simulink model "ModelAgriAuto"  (R2022a)
settings: Solver=FixedStepAuto  StartTime=0.0  StopTime=6240  FixedStep=0.05  MaxStep=0.1  RelTol=1e-3
model workspace (MAT data in the model file):
  PlowHectare = 1.925
values from neighbouring files (symbols this model uses):
  C_rate = 3    [start_function.m]
  Compaction = 0    [start_function.m]
  CyclesIn = CyclesIn+CyclesOut(end)    [start_function.m]
  Degradation = 2    [start_function.m]
  FailRate = 29700000    [start_function.m]
  FieldEff = 0.8    [start_function.m]
  ForceCorrVar = 0.85    [start_function.m]
  Fuel = 3    [start_function.m]
  Mass = 10550    [start_function.m]
  n = n+1    (= 2)    [start_function.m]
  v_field = 5    [start_function.m]
  Weather_crit = 3    [start_function.m]
  WorkingHours = 10    [start_function.m]
undefined symbols (not defined in the file or in its folder): Battery, BatteryNo, Charger, ChargerNo, DField, m, Power, Soil, TractorNo, Year
libraries: simulink x2
(part 1 of 3)
settings Model: Creator=osov0001  LastModifiedBy=osov0001
settings SolverCC: AlgebraicLoopSolver=LineSearch
settings DataIOCC: ExternalInput=[Power, Battery, Charger]  SaveFormat=Array  SaveOutput=off  DSMLogging=off  ReturnWorkspaceOutputs=off
settings DebuggingCC: UnconnectedInputMsg=warning  UnconnectedOutputMsg=warning  UnconnectedLineMsg=warning  SFMachineParentedDataDiag=warning  ArithmeticOperatorsInVariantConditions=warning
settings SFSimCC: SimUseLocalCustomCode=off  CustomCodeUndefinedFunction=UseInterfaceOnly
settings RTWCC: RTWUseLocalCustomCode=off

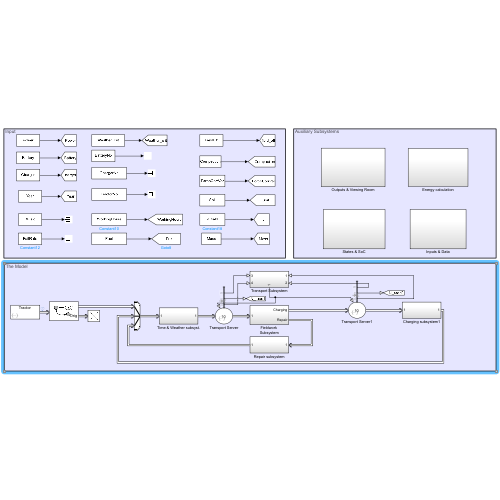
[thumbnail: Simulink's stored preview of the top-level diagram]
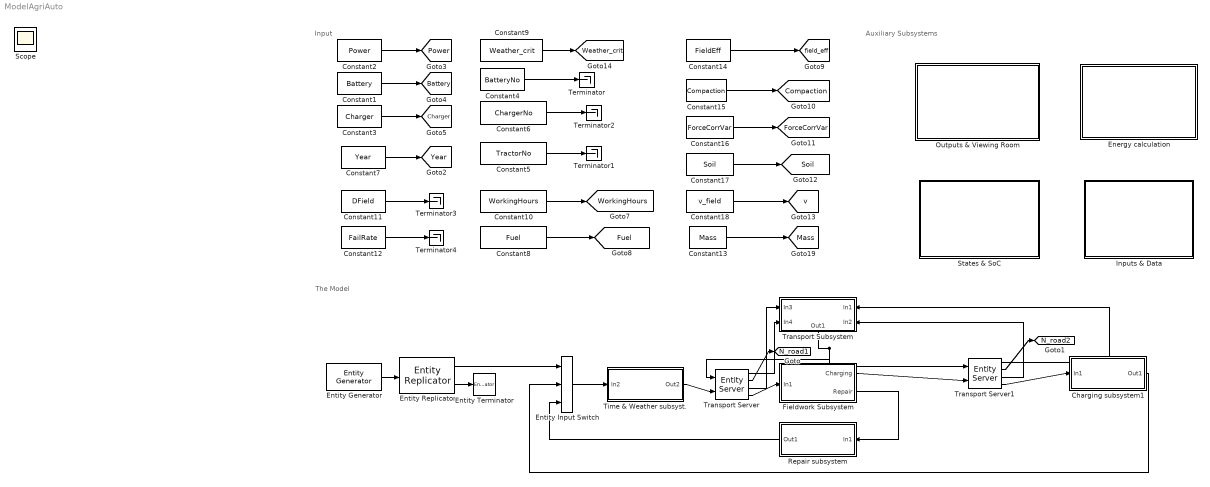
== system ModelAgriAuto ==
  note: The Model
  note: Input
  note: Auxiliary Subsystems
  Charging subsystem1 : Subsystem
  Constant1 : Constant  Value=Battery
  Constant10 : Constant  Value=WorkingHours
  Constant11 : Constant  Value=DField
  Constant12 : Constant  Value=FailRate
  Constant13 : Constant  Value=Mass
  Constant14 : Constant  Value=FieldEff
  Constant15 : Constant  Value=Compaction
  Constant16 : Constant  Value=ForceCorrVar
  Constant17 : Constant  Value=Soil
  Constant18 : Constant  Value=v_field
  Constant2 : Constant  Value=Power
  Constant3 : Constant  Value=Charger
  Constant4 : Constant  Value=BatteryNo
  Constant5 : Constant  Value=TractorNo
  Constant6 : Constant  Value=ChargerNo
  Constant7 : Constant  Value=Year
  Constant8 : Constant  Value=Fuel
  Constant9 : Constant  Value=Weather_crit
  Energy calculation : Subsystem
  Entity Input Switch : EntityInputSwitch  InputPortMessageModes=m,m,m  OutputPortMessageModes=m  NumberInputPorts=3
      settings: InputPortMap=u1,u2,u3
  Entity Generator : EntityGenerator  OutputPortMessageModes=m  Period=inf  GenerateAction=|  AttributeName=SoC|RoadTime|RoF  AttributeInitialValue=1|1|1  EntityType=Structured  EntityTypeName=Tractor
      | entity.SoC=1;
      | entity.RoF=1;
  Entity Replicator : EntityReplicator  InputPortMessageModes=m  OutputPortMessageModes=m,m  ReplicasDepartFrom=Single output port  NumberReplicas=TractorNo  HoldOriginalEntityUntilAllReplicasDepart=on
  Entity Terminator : EntityTerminator  InputPortMessageModes=m
  Fieldwork Subsystem : Subsystem
  Inputs & Data : Subsystem  Tag=INPUTS
  Outputs & Viewing Room : Subsystem
  Repair subsystem : Subsystem
  States & SoC : Subsystem
  Terminator{,1..4} (5 alike) : Terminator
  Time & Weather subsyst. : Subsystem
  Transport Server : EntityServer  InputPortMessageModes=n,m  OutputPortMessageModes=n,n,n,m  Capacity=10  ServiceTimeSource=Signal port  ServiceTimeAttributeName=RoadTime  ServiceCompleteAction=entity.SoC=entity.SoC-0.025;  NumberEntitiesDeparted=on  NumberEntitiesInBlock=on  AverageWait=on
      settings: InputPortMap=u0,u2  OutputPortMap=o0,o1,o4,o9
  Transport Server1 : EntityServer  InputPortMessageModes=n,m  OutputPortMessageModes=n,n,n,m  Capacity=10  ServiceTimeSource=Signal port  ServiceTimeAttributeName=RoadTime  ServiceCompleteAction=entity.SoC=entity.SoC-0.025;  NumberEntitiesDeparted=on  NumberEntitiesInBlock=on  AverageWait=on
      settings: InputPortMap=u0,u2  OutputPortMap=o0,o1,o4,o9
  Transport Subsystem : Subsystem
      settings: PortSchema="{\"entries\":[{\"content\":{\"sides\":[{\"content\":{\"connectorIds\":[\"In1\",\"In2\"]},\"type\":\"ConnectorPlacement.EquallySpacedRectSide\",\"uuid\":\"550b19fe-7368-4b75-be55-a28990181de4\"},{\"content\":{\"connectorIds\":[\"In3\",\"In4\"],\"side\":\"RIGHT\"},\"type\":\"ConnectorPlacement.EquallySpacedRectSide\",\"uuid\":\"f910dc23-d412-48e8-995a-8c291cfed89a\"},{\"content\":{\"connectorIds\":[],\"side\":\"TOP\"},\"type\":\"ConnectorPlacement.EquallySpacedRectSide\",\"uuid\":\"9035d057-4d0f-475c-8836-3d54a9fb5317\"},{\"content\":{\"connectorIds\":[\"Out1\"],\"side\":\"BOTTOM\"},\"type\":\"ConnectorPlacement.EquallySpacedRectSide\",\"uuid\":\"2f36d4ef-6e1b-49a3-b865-e90f10116552\"}]},\"type\":\"ConnectorPlacement.EquallySpacedConnector\",\"uuid\":\"6736081e-50e9-4bc7-8291-962b989661d1\"}],\"packageUris\":[\"http://schema.mathworks.com/mf0/Connector/R2020b\"],\"version\":\"1.0\"}"
  Scope : Scope
  tag scope: Battery=global, Charger=global, Compaction=global, ForceCorrVar=global, Fuel=global, Mass=global, N_road1=global, N_road2=global, Power=global, Soil=global, Weather_crit=global, WorkingHours=global, Year=global, field_eff=global, v=global
  wires:
  Entity Replicator/2 -> Entity Terminator/1
  Entity Generator/1 -> Entity Replicator/1
  Fieldwork Subsystem/1(Charging) -> Transport Server1/2
  Transport Server1/4 -> Charging subsystem1/1(In1)
  Charging subsystem1/1(Out1) -> Entity Input Switch/2
  Repair subsystem/1(Out1) -> Entity Input Switch/3
  Entity Input Switch/1 -> Time & Weather subsyst./1(In2)
  Fieldwork Subsystem/2(Repair) -> Repair subsystem/1(In1)
  Constant1/1 -> [Battery]
  Constant3/1 -> [Charger]
  Constant6/1 -> Terminator2/1
  Constant5/1 -> Terminator1/1
  Constant4/1 -> Terminator/1
  Constant7/1 -> [Year]
  Constant9/1 -> [Weather_crit]
  Transport Server1/3 -> Transport Subsystem/2(In2)
  Transport Server1/1 -> Transport Subsystem/1(In1)
  Entity Replicator/1 -> Entity Input Switch/1
  Transport Server/2 -> [N_road1]
  Transport Server1/2 -> [N_road2]
  Constant10/1 -> [WorkingHours]
  Constant8/1 -> [Fuel]
  Transport Server/4 -> Fieldwork Subsystem/1(In1)
  Constant11/1 -> Terminator3/1
  Time & Weather subsyst./1(Out2) -> Transport Server/2
  Constant2/1 -> [Power]
  Constant12/1 -> Terminator4/1
  Constant13/1 -> [Mass]
  Constant14/1 -> [field_eff]
  Constant15/1 -> [Compaction]
  Constant16/1 -> [ForceCorrVar]
  Constant17/1 -> [Soil]
  Constant18/1 -> [v]
  Transport Subsystem/1(Out1) -> Transport Server/1, Transport Server1/1
  Transport Server/3 -> Transport Subsystem/3(In3)
  Transport Server/1 -> Transport Subsystem/4(In4)

== system ModelAgriAuto/Charging subsystem1 ==
  note: Tid att ladda [h]
  In1 : Inport
  Add3 : Sum  Inputs=+++
  Add4 : Sum
  Add5 : Sum
  Avg queue length : Display
  Avg wait time [h] : Display
  Battery exchange system : Subsystem
  "Charger type and power calculation subsystem " : Subsystem
  Display : DisplayBlock  LabelPosition=Hide  Format=long
  Display2 : Display
  Energy Calculation : Subsystem
  Entity Input Switch1 : EntityInputSwitch  InputPortMessageModes=m,m  OutputPortMessageModes=m
  Entity Output Switch1 : EntityOutputSwitch  InputPortMessageModes=m,m  OutputPortMessageModes=m,m  SwitchingCriterion=From control port  SwitchAttributeName=Attribute1
      settings: InputPortMap=u0,u1
  Entity Queue1 : Queue  InputPortMessageModes=m  OutputPortMessageModes=n,n,m  AverageWait=on  AverageQueueLength=on
      settings: OutputPortMap=o2,o3,o5
  Product1 : Product  Inputs=3
  Product2 : Product
  To Workspace : ToWorkspace  VariableName=TC  SampleTime=1
      settings: Save2DSignal=2-D array (concatenate along first dimension)
  To Workspace1 : ToWorkspace  VariableName=Q_wait_avg  SampleTime=1
  To Workspace3 : ToWorkspace  VariableName=TQ  SampleTime=1
      settings: Save2DSignal=2-D array (concatenate along first dimension)
  Traditional charging/refueling : Subsystem
  Out1 : Outport  VectorParamsAs1DForOutWhenUnconnected=off
  tag scope: Charger_time=global, T_Charge=global
  wires:
  Entity Queue1/3 -> Entity Output Switch1/2
  In1/1 -> Entity Queue1/1
  "Charger type and power calculation subsystem "/1(Charger time) -> [Charger_time]
  Entity Output Switch1/1 -> Traditional charging/refueling/1(In1)
  "Charger type and power calculation subsystem "/2(Charger type) -> Entity Output Switch1/1
  Product1/1 -> Add3/2
  Entity Queue1/1 -> To Workspace1/1, Product1/1, Avg wait time [h]/1  "Avg waiting time [h]"
  Add4/1 -> Display2/1, [T_Charge]
  Entity Queue1/2 -> Avg queue length/1, Product1/2  "Avg queue length [no.]"
  Entity Input Switch1/1 -> Out1/1
  Product2/1 -> Add5/1
  [Charge_no] -> Product1/3
  [Change_no] -> Product2/1
  Traditional charging/refueling/4(Charge time) -> Add5/2
  Add5/1 -> Add4/2, To Workspace/1
  Add3/1 -> To Workspace3/1, Add4/1
  Traditional charging/refueling/2(Queue time) -> Add3/3
  Traditional charging/refueling/1(Out1) -> Entity Input Switch1/1
  Traditional charging/refueling/3(Entities departed) -> Energy Calculation/1(In1)
  Entity Output Switch1/2 -> Battery exchange system/1(In2)
  Battery exchange system/1(Out2) -> Entity Input Switch1/2
  Battery exchange system/2(Out1) -> Product2/2
  Battery exchange system/3(Out3) -> Add3/1

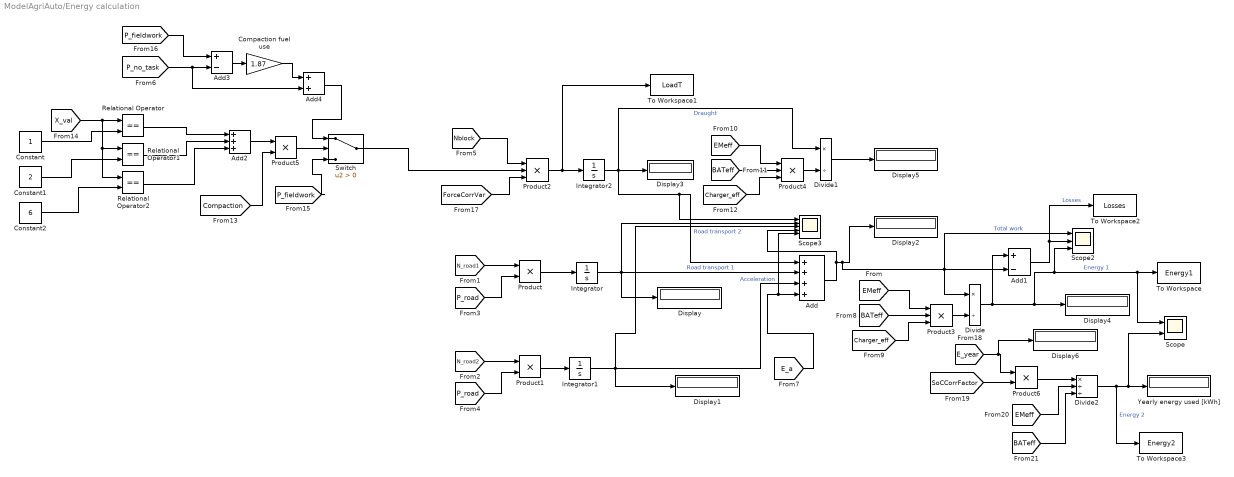
== system ModelAgriAuto/Energy calculation ==
  Add : Sum  Inputs=++++
  Add1 : Sum  Inputs=+-
  Add2 : Sum  Inputs=+++
  Add3 : Sum  Inputs=+-
  Add4 : Sum
  Compaction fuel use : Gain  Gain=1.87
  Constant : Constant
  Constant1 : Constant  Value=2
  Constant2 : Constant  Value=6
  Display{,1..6} (7 alike) : Display
  Divide : Product  Inputs=*/
  Divide1 : Product  Inputs=*/
  Divide2 : Product  Inputs=*//
  Integrator : Integrator
  Integrator1 : Integrator
  Integrator2 : Integrator
  Product{,1,5..6} (4 alike) : Product
  Product2 : Product  Inputs=3
  Product3 : Product  Inputs=3
  Product4 : Product  Inputs=3
  Relational Operator : RelationalOperator  Operator===  OutDataTypeStr=boolean  RndMeth=Simplest  InputSameDT=off
  Relational Operator1 : RelationalOperator  Operator===  OutDataTypeStr=boolean  RndMeth=Simplest  InputSameDT=off
  Relational Operator2 : RelationalOperator  Operator===  OutDataTypeStr=boolean  RndMeth=Simplest  InputSameDT=off
  Scope : Scope  NumInputPorts=2
  Scope2 : Scope  NumInputPorts=3
  Scope3 : Scope  NumInputPorts=5
  Switch : Switch  Criteria=u2 > Threshold  SaturateOnIntegerOverflow=off  InputSameDT=off
  To Workspace : ToWorkspace  VariableName=Energy1  SampleTime=1
  To Workspace1 : ToWorkspace  VariableName=LoadT  SampleTime=0.5
      settings: Save2DSignal=2-D array (concatenate along first dimension)
  To Workspace2 : ToWorkspace  VariableName=Losses  SampleTime=1
  To Workspace3 : ToWorkspace  VariableName=Energy2  SampleTime=1
  Yearly energy used [kWh] : Display
  wires:
  [N_road1] -> Product/1
  [P_road] -> Product/2
  [P_road] -> Product1/2
  [N_road2] -> Product1/1
  Product/1 -> Integrator/1
  Product1/1 -> Integrator1/1
  Integrator/1 -> Add/2, Scope3/2, Display/1  "Road transport 1"
  Integrator1/1 -> Add/3, Display1/1, Scope3/3  "Road transport 2"
  Add/1 -> Display2/1, Add1/2, Divide/1, Scope2/1, Scope3/4  "Total work"
  [Nblock] -> Product2/1
  [E_a] -> Scope3/5, Add/4  "Acceleration"
  Divide/1 -> Add1/1, Scope2/3, Scope/1, To Workspace/1, Display4/1  "Energy 1"
  [Charger_eff] -> Product3/3
  [BATeff] -> Product3/2
  [EMeff] -> Product3/1
  Product3/1 -> Divide/2
  [Charger_eff] -> Product4/3
  [EMeff] -> Product4/1
  Product4/1 -> Divide1/2
  [BATeff] -> Product4/2
  Integrator2/1 -> Display3/1, Scope3/1, Add/1, Divide1/1  "Draught"
  Divide1/1 -> Display5/1
  Product2/1 -> Integrator2/1, To Workspace1/1
  Add1/1 -> Scope2/2, To Workspace2/1  "Losses"
  Relational Operator/1 -> Add2/1
  Relational Operator1/1 -> Add2/2
  Relational Operator2/1 -> Add2/3
  [X_val] -> Relational Operator2/1, Relational Operator1/1, Relational Operator/1
  Constant/1 -> Relational Operator/2
  Constant1/1 -> Relational Operator1/2
  Constant2/1 -> Relational Operator2/2
  Add2/1 -> Product5/1
  [Compaction] -> Product5/2
  Product5/1 -> Switch/2
  [P_fieldwork] -> Switch/3
  Switch/1 -> Product2/2
  [P_fieldwork] -> Add3/1
  [P_no_task] -> Add4/2, Add3/2
  Add3/1 -> Compaction fuel use/1
  Compaction fuel use/1 -> Add4/1
  Add4/1 -> Switch/1
  [ForceCorrVar] -> Product2/3
  Divide2/1 -> To Workspace3/1, Scope/2, Yearly energy used [kWh]/1  "Energy 2"
  Product6/1 -> Divide2/1
  [BATeff] -> Divide2/3
  [E_year] -> Display6/1, Product6/1
  [EMeff] -> Divide2/2
  [SoCCorrFactor] -> Product6/2

== system ModelAgriAuto/Fieldwork Subsystem ==
  In1 : Inport
  Active working time [days] : Display
  Entity Output Switch : EntityOutputSwitch  InputPortMessageModes=m  OutputPortMessageModes=m,m  SwitchingCriterion=From attribute  SwitchAttributeName=entity.RoF
  Entity Gate : EntityGate  InputPortMessageModes=m,m  OutputPortMessageModes=m  OpenGateAtSimulationStart=on
  Entity Queue : Queue  InputPortMessageModes=m  OutputPortMessageModes=n,n,m  Capacity=10  NumberEntitiesDeparted=on  AverageWait=on
      settings: OutputPortMap=o0,o2,o5
  Failure check : EntityServer  InputPortMessageModes=m  OutputPortMessageModes=m  Capacity=1  ServiceTimeValue=0.01  ServiceCompleteAction=|
      | M=(FailRate);
      | x=randi (M);
      | 
      | % if-loop determined by Rate- of-failure
      | if x>=M;
      |     entity.RoF=2;
      | else
      |     entity.RoF=1;
      | end
  Field Subsystem : Subsystem
  "Fieldwork time subsystem " : Subsystem
  FieldworkServer : EntityServer  InputPortMessageModes=n,m  OutputPortMessageModes=n,n,n,m  Capacity=10  ServiceTimeSource=Signal port  ServiceTimeValue=3.843  NumberEntitiesDeparted=on  NumberEntitiesInBlock=on  AverageWait=on
      settings: InputPortMap=u0,u2  OutputPortMap=o0,o1,o4,o9
  Message Send : Send  OutputPortMessageModes=m
  No. of tractor-trips : Display
  Null Server : EntityServer  InputPortMessageModes=m  OutputPortMessageModes=n,m  Capacity=1  ServiceTimeValue=0.0001  NumberEntitiesDeparted=on
      settings: OutputPortMap=o0,o9
  Product : Product
  Product1 : Product
  Saturation : Saturate  UpperLimit=WorkingHours  LowerLimit=0
  Scope : Scope
  To Workspace : ToWorkspace  VariableName=Hectares  SampleTime=1
  To Workspace1 : ToWorkspace  VariableName=Field  SampleTime=1
  To Workspace2 : ToWorkspace  VariableName=Task  SampleTime=1
  To Workspace3 : ToWorkspace  VariableName=WorkTime  SampleTime=1
  h to days : Gain  Gain=1/24
  Charging : Outport  VectorParamsAs1DForOutWhenUnconnected=off
  Repair : Outport  Port=2  VectorParamsAs1DForOutWhenUnconnected=off
  tag scope: Field=global, Nblock=global, T_Wait=global, T_Work=global, Trips=global
  wires:
  In1/1 -> Null Server/1
  FieldworkServer/3 -> Product/1
  Null Server/2 -> Entity Queue/1
  Field Subsystem/4(Out5) -> To Workspace/1  "H out total"
  Field Subsystem/1(Out2) -> Message Send/1
  Field Subsystem/3(Out4) -> To Workspace2/1  "Task number"
  Message Send/1 -> Entity Gate/1
  Field Subsystem/2(Out3) -> [Field], To Workspace1/1  "Field number"
  FieldworkServer/1 -> Product/2
  Null Server/1 -> [Trips], No. of tractor-trips/1
  Product1/1 -> [T_Wait]
  Entity Queue/1 -> Product1/2
  Entity Queue/2 -> Product1/1
  Entity Queue/3 -> Entity Gate/2
  FieldworkServer/2 -> [Nblock], Field Subsystem/1(N_block)
  Entity Output Switch/1 -> FieldworkServer/2
  Entity Output Switch/2 -> Repair/1
  Failure check/1 -> Entity Output Switch/1
  Entity Gate/1 -> Failure check/1
  Product/1 -> h to days/1, [T_Work], To Workspace3/1
  h to days/1 -> Active working time [days]/1
  "Fieldwork time subsystem "/1(Out1) -> Saturation/1
  Saturation/1 -> Scope/1, FieldworkServer/1
  FieldworkServer/4 -> Charging/1

== system ModelAgriAuto/Inputs & Data ==
  note: Fuel & Driveline inputs
  note: Weather inputs
  note: Charger inputs
  note: Field, soil and crop rotation inputs
  Battery and driveline inputs : Subsystem
  Charging inputs : Subsystem
  Field inputs : Subsystem
  "Fuel/mode selection " : Subsystem
  Weather Inputs : Subsystem

== system ModelAgriAuto/Outputs & Viewing Room ==
  note: Time distribution
  note: Periods:
      |
      | Spring period: 0 - 1512 h
      |
      | Growing period: 1513 - 2208 h
      |
      | Summer period: 2209 - 2976 h
      |
      | Growing and harvest period: 2978 - 4104 h
      |
      | Fall period: 4105-5600 h
  note: Operation order:
      |
      | 1: -
      | 2: Harrow / Harvning
      | 3: Fert. Spreading / Gödsling
      | 4: Harrow / Harvning
      | 5: Sowing / Sådd
      | 6: Roller packing / Vältning
      | ------
      | 7: Fert. Spreading / Gödsling
      | 8: Fert. Spreading / Gödsling
      | 9: Pesticide Spreading / Växtskydd
      | ------
      | (Harvest / Skörd)
      | 10: Cultivation / Stubbning
      | 11: Cultivation / Sladdning
      | 12: Roller packing / Vältning
      | 13: Fert. Spreading / Gödsling
      | 14: Harrow / Harvning
      | 15: Harrow / Harvning
      | 16: Sowing / Sådd
      | 17: Plowing / Plöjning
  Active time in field [days] : DisplayBlock  LabelPosition=Hide  Format=long
  Dashboard Scope : DashboardScope  Ymin=0  Ymax=100
  Favourable weather [%] : DisplayBlock  LabelPosition=Hide  Format=long
  No. of charges : DisplayBlock  LabelPosition=Hide  Format=long
  No. of repairs : DisplayBlock  LabelPosition=Hide  Format=long
  No. of trips : DisplayBlock  LabelPosition=Hide  Format=long
  Rate of failure [%] : DisplayBlock  LabelPosition=Hide  Format=long
  Time Management Subsystem : Subsystem
  Time required (alt) [days/yr] : DisplayBlock  LabelPosition=Hide  Format=long
  Yearly energy consumption [kWh] : DisplayBlock  LabelPosition=Hide  Format=shortE

== system ModelAgriAuto/Repair subsystem ==
  In1 : Inport
  Display1 : Display
  Gain : Gain  Gain=100
  No. of repairs : Display
  Product1 : Product  Inputs=**
  Product2 : Product  Inputs=*/
  Repair : EntityServer  InputPortMessageModes=n,m  OutputPortMessageModes=n,m  Capacity=1  ServiceTimeSource=Signal port  ServiceTimeValue=24  NumberEntitiesDeparted=on
      settings: InputPortMap=u0,u2  OutputPortMap=o0,o9
  Repair time : Constant  Value=24
  Out1 : Outport  VectorParamsAs1DForOutWhenUnconnected=off
  tag scope: RoF=global, T_Repair=global
  wires:
  Repair/1 -> Product2/1, Product1/2, No. of repairs/1
  In1/1 -> Repair/2
  Repair/2 -> Out1/1
  Product2/1 -> [RoF]
  [Trips] -> Product2/2
  Repair time/1 -> Repair/1, Product1/1
  Product1/1 -> [T_Repair]
  Gain/1 -> Display1/1
  [RoF] -> Gain/1

== system ModelAgriAuto/States & SoC ==
  note: NOTE: Soc does not work for BES
  Add : Sum
  Add1 : Sum
  Add2 : Sum
  Chart : Stateflow chart  TreatAsAtomicUnit=on
  Divide : Product  Inputs=*/
  Gain : Gain
  Integrator : Integrator  InitialCondition=1  LimitOutput=on  UpperSaturationLimit=1  LowerSaturationLimit=0
  Product : Product
  Product1 : Product
  Scope : Scope  NumInputPorts=2
  Scope1 : Scope  NumInputPorts=3
  Sequence Viewer : MessageViewer  Commented=on  History=1000
  To Workspace : ToWorkspace  VariableName=State  SampleTime=-1
  To Workspace1 : ToWorkspace  VariableName=SoCState  SampleTime=-1
  tag scope: State=global
  wires:
  [Nblock] -> Chart/1(Nblock)
  [BESblock] -> Chart/3(BESblock)
  [CCblock] -> Chart/2(CCblock)
  [N_road1] -> Add2/1
  [N_road2] -> Add2/2
  [Charger] -> Product/1
  [P_road] -> Chart/6(P_road)
  [P_fieldwork] -> Chart/5(P_fieldwork)
  Product/1 -> Chart/7(Charger)
  [Charger_eff] -> Product/2
  Chart/1(SoCchange) -> Divide/1
  Integrator/1 -> To Workspace1/1, Scope/1  "SoC"
  [Battery] -> Product1/1
  [SOC] -> Product1/2
  Divide/1 -> Integrator/1
  Chart/2(State) -> To Workspace/1, [State], Scope/2  "State"
  [CCblock] -> Add/1
  [BESblock] -> Add/2
  [N_road1] -> Add1/1
  [N_road2] -> Add1/2
  Add/1 -> Scope1/3  "Charging"
  Add1/1 -> Scope1/2  "Transport"
  [Nblock] -> Gain/1  "Fieldwork"
  Product1/1 -> Divide/2
  Gain/1 -> Scope1/1  "Fieldwork"
  Add2/1 -> Chart/4(Nroad_1)

== system ModelAgriAuto/Time & Weather subsyst. ==
  In2 : Inport
  Driver work-time subsystem : Subsystem
  Weather & schedule subsystem : Subsystem
  Out2 : Outport  VectorParamsAs1DForOutWhenUnconnected=off
  wires:
  In2/1 -> Driver work-time subsystem/1(In1)
  Driver work-time subsystem/1(Out1) -> Weather & schedule subsystem/1(In1)
  Weather & schedule subsystem/1(Out1) -> Out2/1

== system ModelAgriAuto/Transport Subsystem ==
  note: Road Forces & Transport time
  In1 : Inport
  In2 : Inport  Port=2
  In3 : Inport  Port=3
  In4 : Inport  Port=4
  Add1 : Sum
  Add2 : Sum
  Constant1 : Constant  Value=0.03333333
  Demux : Demux  Outputs=12
  Distance Values Switch : MultiPortSwitch  Inputs=12  SaturateOnIntegerOverflow=off  InputSameDT=off
  Divide1 : Product  Inputs=*/
  Divide3 : Product  Inputs=*/
  Divide5 : Product  Inputs=/*
  Gain1 : Gain  Gain=2
  Gain2 : Gain  Gain=3.6
  Mean road speed : Display
  Memory : Memory  InitialCondition=1
  No task transport time : Constant  Value=0.1
  Product : Product
  Product2 : Product
  Road forces : Subsystem
  Scope : Scope  NumInputPorts=2
  Scope2 : Scope
  Scope4 : Scope
  Sum : Sum  Inputs=-+
  Switch : Switch  Criteria=u2 > Threshold  SaturateOnIntegerOverflow=off  InputSameDT=off
  To Workspace : ToWorkspace  VariableName=TransportTime  SampleTime=1
  Transport time [h] : Display
  acc distance [km] 1 : Constant  Value=0.29
  Out1 : Outport
  tag scope: T_Transport=global, T_travel=global, v_road_actual=global
  wires:
  [v_road_actual] -> Mean road speed/1, Divide1/2
  Divide1/1 -> Switch/1, Scope4/1, Transport time [h]/1, [T_travel]
  [Field] -> Distance Values Switch/1, Scope/2
  [Field_distance] -> Demux/1
  Demux/12 -> Distance Values Switch/13
  Demux/11 -> Distance Values Switch/12
  Demux/10 -> Distance Values Switch/11
  Demux/9 -> Distance Values Switch/10
  Demux/8 -> Distance Values Switch/9
  Demux/7 -> Distance Values Switch/8
  Demux/6 -> Distance Values Switch/7
  Demux/5 -> Distance Values Switch/6
  Demux/4 -> Distance Values Switch/5
  Demux/3 -> Distance Values Switch/4
  Demux/2 -> Distance Values Switch/3
  Demux/1 -> Distance Values Switch/2
  [a] -> Road forces/2(a)
  [m] -> Road forces/1("m ")
  In1/1 -> Road forces/3("N_block "), Product/1
  Add2/1 -> [T_Transport], To Workspace/1
  In2/1 -> Product/2
  [v_road] -> Memory/1
  Gain2/1 -> Divide3/2
  Distance Values Switch/1 -> Scope/1, Sum/2, Divide5/2, Divide1/1
  Constant1/1 -> Add1/2
  Add1/1 -> Divide5/1
  acc distance [km] 1/1 -> Gain1/1
  Sum/1 -> Divide3/1
  Divide3/1 -> Add1/1
  Gain1/1 -> Sum/1
  Divide5/1 -> [v_road_actual]
  Memory/1 -> Gain2/1
  [X_val] -> Switch/2
  Switch/1 -> Scope2/1, Out1/1
  No task transport time/1 -> Switch/3
  In3/1 -> Product2/1
  In4/1 -> Product2/2
  Product2/1 -> Add2/2
  Product/1 -> Add2/1

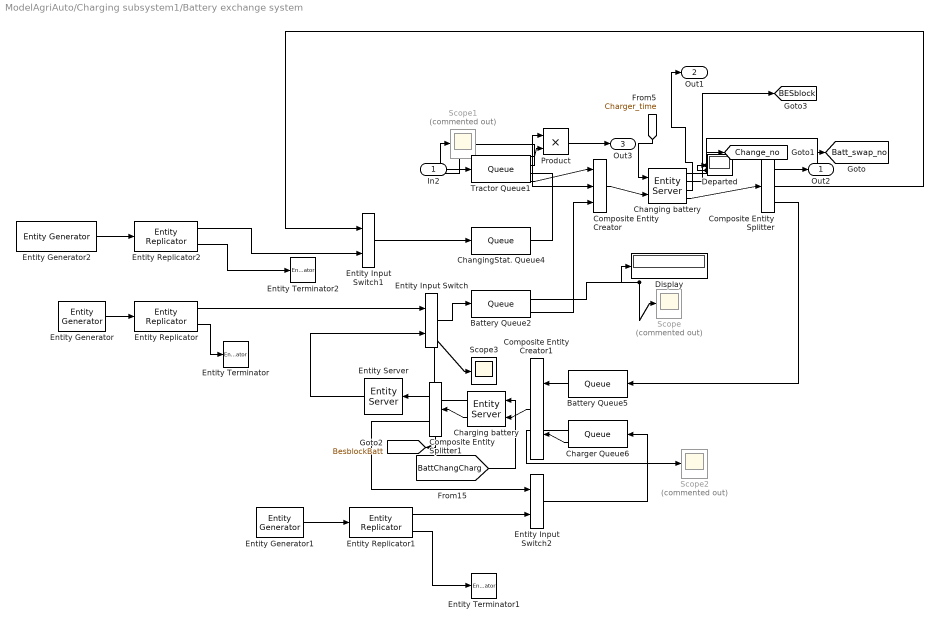
== system ModelAgriAuto/Charging subsystem1/Battery exchange system ==
  In2 : Inport
  Battery Queue2 : Queue  InputPortMessageModes=m  OutputPortMessageModes=n,m  NumberEntitiesInBlock=on
      settings: OutputPortMap=o1,o5
  Battery Queue5 : Queue  InputPortMessageModes=m  OutputPortMessageModes=m
  Changing battery : EntityServer  InputPortMessageModes=n,m  OutputPortMessageModes=n,n,n,m  Capacity=10  ServiceTimeSource=Signal port  NumberEntitiesDeparted=on  NumberEntitiesInBlock=on  AverageWait=on
      settings: InputPortMap=u0,u2  OutputPortMap=o0,o1,o4,o9
  ChangingStat. Queue4 : Queue  InputPortMessageModes=m  OutputPortMessageModes=m
  Charger Queue6 : Queue  InputPortMessageModes=m  OutputPortMessageModes=n,m  NumberEntitiesInBlock=on
      settings: OutputPortMap=o1,o5
  Charging battery : EntityServer  InputPortMessageModes=n,m  OutputPortMessageModes=n,m  Capacity=10  ServiceTimeSource=Signal port  NumberEntitiesInBlock=on
      settings: InputPortMap=u0,u2  OutputPortMap=o1,o9
  Composite Entity Creator : CompositeEntityCreator  InputPortMessageModes=m,m,m  OutputPortMessageModes=m  NumberInputPorts=3  EntityTypeName=BatteryChangingStation  InputEntityName=Tractor|ChangingStation|Battery
      settings: InputPortMap=u0,u1,u2
  Composite Entity Creator1 : CompositeEntityCreator  InputPortMessageModes=m,m  OutputPortMessageModes=m  EntityTypeName=Combined
      settings: InputPortMap=u0,u1
  Composite Entity Splitter : CompositeEntitySplitter  InputPortMessageModes=m  OutputPortMessageModes=m,m,m  NumberOutputPorts=3
      settings: OutputPortMap=o0,o1,o2
  Composite Entity Splitter1 : CompositeEntitySplitter  InputPortMessageModes=m  OutputPortMessageModes=m,m
      settings: OutputPortMap=o0,o1
  Departed : Display
  Display : Display
  Entity Input Switch : EntityInputSwitch  InputPortMessageModes=m,m  OutputPortMessageModes=m
  Entity Input Switch1 : EntityInputSwitch  InputPortMessageModes=m,m  OutputPortMessageModes=m
  Entity Input Switch2 : EntityInputSwitch  InputPortMessageModes=m,m  OutputPortMessageModes=m
  Entity Generator : EntityGenerator  OutputPortMessageModes=m  Period=99999999  AttributeName=SoC|Cycle  AttributeInitialValue=1|1  EntityType=Structured  EntityTypeName=Battery
  Entity Generator1 : EntityGenerator  OutputPortMessageModes=m  Period=99999999  AttributeName=data  EntityType=Structured  EntityTypeName=Charger
  Entity Generator2 : EntityGenerator  OutputPortMessageModes=m  Period=99999999  AttributeName=data  EntityType=Structured  EntityTypeName=ChangingStation
  Entity Replicator : EntityReplicator  InputPortMessageModes=m  OutputPortMessageModes=m,m  ReplicasDepartFrom=Single output port  NumberReplicas=BatteryNo+TractorNo
  Entity Replicator1 : EntityReplicator  InputPortMessageModes=m  OutputPortMessageModes=m,m  ReplicasDepartFrom=Single output port  NumberReplicas=ChargerNo
  Entity Replicator2 : EntityReplicator  InputPortMessageModes=m  OutputPortMessageModes=m,m  ReplicasDepartFrom=Single output port  NumberReplicas=ChangeNo
  Entity Server : EntityServer  InputPortMessageModes=m  OutputPortMessageModes=m  Capacity=1  ServiceTimeValue=0.001  ServiceCompleteAction=entity.Cycle=entity.Cycle + 1;
  Entity Terminator : EntityTerminator  InputPortMessageModes=m
  Entity Terminator1 : EntityTerminator  InputPortMessageModes=m
  Entity Terminator2 : EntityTerminator  InputPortMessageModes=m
  Product : Product
  Scope : Scope  Commented=on
  Scope1 : Scope  Commented=on
  Scope2 : Scope  Commented=on
  Scope3 : Scope
  Tractor Queue1 : Queue  InputPortMessageModes=m  OutputPortMessageModes=n,n,n,m  NumberEntitiesDeparted=on  NumberEntitiesInBlock=on  AverageWait=on
      settings: OutputPortMap=o0,o1,o2,o5
  Out2 : Outport
  Out1 : Outport  Port=2
  Out3 : Outport  Port=3
  tag scope: BESblock=global, Batt_swap_no=global, BesblockBatt=global, Change_no=global
  wires:
  Entity Replicator/1 -> Entity Input Switch/1
  Entity Generator1/1 -> Entity Replicator1/1
  Entity Replicator1/1 -> Entity Input Switch2/2
  Entity Replicator1/2 -> Entity Terminator1/1
  Entity Replicator/2 -> Entity Terminator/1
  Entity Generator/1 -> Entity Replicator/1
  In2/1 -> Tractor Queue1/1
  Tractor Queue1/4 -> Composite Entity Creator/1
  Composite Entity Splitter/1 -> Out2/1
  Entity Replicator2/2 -> Entity Terminator2/1
  Entity Generator2/1 -> Entity Replicator2/1
  Entity Replicator2/1 -> Entity Input Switch1/2
  Battery Queue2/2 -> Composite Entity Creator/3
  Composite Entity Creator/1 -> Changing battery/2
  Changing battery/4 -> Composite Entity Splitter/1
  Entity Input Switch/1 -> Battery Queue2/1
  Composite Entity Splitter/3 -> Battery Queue5/1
  Entity Input Switch1/1 -> ChangingStat. Queue4/1
  ChangingStat. Queue4/1 -> Composite Entity Creator/2
  Composite Entity Splitter/2 -> Entity Input Switch1/1
  Battery Queue5/1 -> Composite Entity Creator1/1
  Charger Queue6/2 -> Composite Entity Creator1/2
  Composite Entity Creator1/1 -> Charging battery/2
  Charging battery/2 -> Composite Entity Splitter1/1
  Composite Entity Splitter1/1 -> Entity Server/1
  Entity Input Switch2/1 -> Charger Queue6/1
  Composite Entity Splitter1/2 -> Entity Input Switch2/1
  Changing battery/1 -> [Batt_swap_no], [Change_no], Departed/1
  Changing battery/2 -> [BESblock]
  Changing battery/3 -> Out1/1
  Tractor Queue1/3 -> Product/1
  Tractor Queue1/1 -> Product/2
  Product/1 -> Out3/1
  [Charger_time] -> Changing battery/1
  [BattChangCharg] -> Charging battery/1
  Battery Queue2/1 -> Scope/1, Display/1
  Charger Queue6/1 -> Scope2/1
  Tractor Queue1/2 -> Scope1/1
  Entity Server/1 -> Entity Input Switch/2
  Charging battery/1 -> Scope3/1, [BesblockBatt]

== system ModelAgriAuto/Charging subsystem1/Charger type and power calculation subsystem  ==
  note: Battery exchange system charger info
  note: Charger info
  note: 1=Conv charging
      | 2=Battery change
  note: de Afonseca (2018)
  "Battery change charger time display " : Display
  Battery changing time [h] : Constant  Value=0.16667
  Clock : Clock
  Constant : Constant
  Display : Display
  Divide : Product  Inputs=**/
  Divide1 : Product  Inputs=**/
  Divide3 : Product  Inputs=*/
  Divide4 : Product  Inputs=**
  Integrator : Integrator
  Message Send : Send  OutputPortMessageModes=m
  Multiport Switch2 : MultiPortSwitch  Inputs=2  SaturateOnIntegerOverflow=off  InputSameDT=off
  Product1 : Product
  Product3 : Product
  Scope2 : Scope
  Charger time : Outport  VectorParamsAs1DForOutWhenUnconnected=off
  Charger type : Outport  Port=2  VectorParamsAs1DForOutWhenUnconnected=off
  tag scope: BattChangCharg=global, Charger_type=global, SoCCorrFactor=global
  wires:
  [P_charger] -> Product3/1
  Divide4/1 -> Divide/1
  [Charger_eff] -> Product3/2
  Product3/1 -> Divide/3
  Multiport Switch2/1 -> Charger time/1
  Message Send/1 -> Charger type/1
  [P_charger_swap] -> Product1/1
  [ChargerChoice] -> [Charger_type], Message Send/1, Multiport Switch2/1
  Divide/1 -> Multiport Switch2/2
  Battery changing time [h]/1 -> Multiport Switch2/3
  [Battery_size] -> Divide1/1
  Product1/1 -> Divide1/3
  Divide1/1 -> [BattChangCharg], "Battery change charger time display "/1
  [Charger_eff] -> Product1/2
  Clock/1 -> Divide3/2
  Integrator/1 -> Divide3/1
  Divide3/1 -> Scope2/1, [SoCCorrFactor], Display/1
  [SOC] -> Divide4/2
  [Battery_size] -> Divide4/1
  [SOC] -> Divide1/2
  [SoC_Frac] -> Integrator/1
  Constant/1 -> Divide/2

== system ModelAgriAuto/Charging subsystem1/Energy Calculation ==
  In1 : Inport
  Add : Sum
  Divide : Product  Inputs=**/
  Divide1 : Product  Inputs=*/*
  Multiport Switch2 : MultiPortSwitch  Inputs=2  SaturateOnIntegerOverflow=off  InputSameDT=off
  No of total charges : Display
  To Workspace1 : ToWorkspace  VariableName=ChargeNo  SampleTime=1
      settings: Save2DSignal=2-D array (concatenate along first dimension)
  tag scope: Charge_no=global, E_year=global
  wires:
  [EstBat] -> Divide1/1, Divide/2
  [Charger_eff] -> Divide1/2, Divide/3
  Divide/1 -> Add/1
  [Charge_no] -> To Workspace1/1, No of total charges/1
  Add/1 -> [E_year]
  [Batt_swap_no] -> Divide1/3
  Divide1/1 -> Add/2
  [Change_no] -> Multiport Switch2/3
  [Charger_type] -> Multiport Switch2/1
  Multiport Switch2/1 -> [Charge_no]
  In1/1 -> Divide/1, Multiport Switch2/2

== system ModelAgriAuto/Charging subsystem1/Traditional charging//refueling ==
  note: Charger load calculation
  note: Charger creation event
  In1 : Inport
  Add : Sum  Inputs=+++
  Add1 : Sum  Inputs=+++
  Add2 : Sum  Inputs=+++
  Add3 : Sum
  Amount available : Scope
  Amount in use : Scope
  Charger Acquirer : EntityResourceAcquirer  InputPortMessageModes=m  OutputPortMessageModes=n,n,m  ResourceName=Charger  NumberEntitiesDeparted=on  AverageWait=on
      settings: OutputPortMap=o0,o2,o3
  Charger Server1 : EntityServer  InputPortMessageModes=n,m  OutputPortMessageModes=n,n,n,m  Capacity=1  ServiceTimeSource=Signal port  ServiceCompleteAction=entity.SoC=1;  NumberEntitiesDeparted=on  NumberEntitiesInBlock=on  AverageWait=on
      settings: InputPortMap=u0,u2  OutputPortMap=o0,o1,o4,o9
  Charger Server2 : EntityServer  InputPortMessageModes=n,m  OutputPortMessageModes=n,n,n,m  Capacity=1  ServiceTimeSource=Signal port  ServiceCompleteAction=entity.SoC=1;  NumberEntitiesDeparted=on  NumberEntitiesInBlock=on  AverageWait=on
      settings: InputPortMap=u0,u2  OutputPortMap=o0,o1,o4,o9
  Charger Server3 : EntityServer  InputPortMessageModes=n,m  OutputPortMessageModes=n,n,n,m  Capacity=1  ServiceTimeSource=Signal port  ServiceCompleteAction=entity.SoC=1;  NumberEntitiesDeparted=on  NumberEntitiesInBlock=on  AverageWait=on
      settings: InputPortMap=u0,u2  OutputPortMap=o0,o1,o4,o9
  Charger releaser : EntityResourceReleaser  InputPortMessageModes=m  OutputPortMessageModes=m  ResourceToRelease=Selected  ResourceName=Charger
  Entity Input Switch : EntityInputSwitch  InputPortMessageModes=m,m,m  OutputPortMessageModes=m  NumberInputPorts=3
      settings: InputPortMap=u1,u2,u3
  Entity Output Switch : EntityOutputSwitch  InputPortMessageModes=m  OutputPortMessageModes=m,m,m  NumberOutputPorts=3  SwitchAttributeName=Attribute1
      settings: OutputPortMap=o0,o1,o2
  Gain : Gain
  Message Send1 : Send  OutputPortMessageModes=m
  No. of chargers : Constant  Value=ChargerNo  SampleTime=100000000
  Product{3..7} (5 alike) : Product
  Resource Pool : EntityResourcePool  InputPortMessageModes=m  ResourceName=Charger  ResourceAmountSource=Change amount through control port  ResourceAmount=1  InitialResourceAmount=0  AmountInUse=on  AverageUtilization=on  AmountAvailable=on
      settings: OutputPortMap=o0,o1,o2
  Scope : Scope
  To Workspace4 : ToWorkspace  VariableName=LoadC  SampleTime=1
      settings: Save2DSignal=2-D array (concatenate along first dimension)
  To Workspace5 : ToWorkspace  VariableName=Charge_use  SampleTime=-1
      settings: Save2DSignal=2-D array (concatenate along first dimension)
  "Utilization, average " : Display
  Out1 : Outport
  Queue time : Outport  Port=2
  Entities departed : Outport  Port=3
  Charge time : Outport  Port=4
  tag scope: CCblock=global
  wires:
  Product3/1 -> Queue time/1
  Charger releaser/1 -> Out1/1
  [Charger_time] -> Charger Server1/1
  Charger Server1/4 -> Entity Input Switch/1
  Entity Output Switch/3 -> Charger Server3/2
  Entity Output Switch/2 -> Charger Server2/2
  Charger Server1/3 -> Product4/1
  Charger Server3/4 -> Entity Input Switch/3
  Charger Acquirer/1 -> Product3/2
  Charger Server2/3 -> Product5/2
  Charger Server1/1 -> Product4/2, Add/1
  [Charger_time] -> Charger Server3/1
  Product4/1 -> Add2/1
  Charger Server3/1 -> Add/3, Product6/2
  [Charger_time] -> Charger Server2/1
  Charger Server2/4 -> Entity Input Switch/2
  Entity Output Switch/1 -> Charger Server1/2
  Product6/1 -> Add2/3
  In1/1 -> Charger Acquirer/1
  Charger Acquirer/3 -> Entity Output Switch/1
  Charger Server2/1 -> Add/2, Product5/1
  Product5/1 -> Add2/2
  Charger Server3/3 -> Product6/1
  Entity Input Switch/1 -> Charger releaser/1
  Charger Acquirer/2 -> Product3/1
  [Charger] -> Product7/1
  Add/1 -> Entities departed/1
  Add2/1 -> Charge time/1
  Resource Pool/1 -> Gain/1, Amount in use/1
  Resource Pool/3 -> Amount available/1
  No. of chargers/1 -> Message Send1/1
  Message Send1/1 -> Resource Pool/1
  Gain/1 -> To Workspace5/1
  Resource Pool/2 -> "Utilization, average "/1  "Avg. Utilization [%]"
  [BesblockBatt] -> Add3/2
  [CCblock] -> Add3/1
  Add3/1 -> Product7/2
  Charger Server2/2 -> Add1/2
  Charger Server3/2 -> Add1/3
  Charger Server1/2 -> Add1/1
  Add1/1 -> [CCblock]
  Product7/1 -> Scope/1, To Workspace4/1

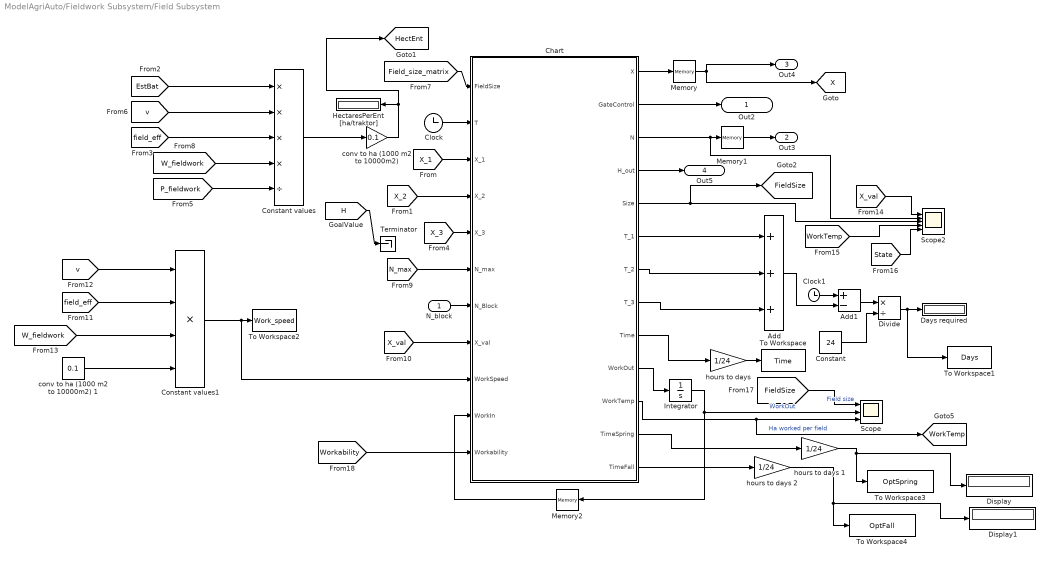
== system ModelAgriAuto/Fieldwork Subsystem/Field Subsystem ==
  N_block : Inport
  Add : Sum  Inputs=+++
  Add1 : Sum  Inputs=+-
  Chart : Stateflow chart  TreatAsAtomicUnit=on
  Clock : Clock
  Clock1 : Clock
  Constant : Constant  Value=24
  Constant values : Product  Inputs=****/
  Constant values1 : Product  Inputs=****
  Days required : Display
  Display : Display
  Display1 : Display
  Divide : Product  Inputs=*/
  HectaresPerEnt [ha/traktor] : Display
  Integrator : Integrator
  Memory : Memory  InitialCondition=1
  Memory1 : Memory  InitialCondition=1
  Memory2 : Memory  InitialCondition=1
  Scope : Scope  NumInputPorts=3
  Scope2 : Scope  NumInputPorts=5
  Terminator : Terminator
  To Workspace : ToWorkspace  VariableName=Time  SampleTime=1
      settings: Save2DSignal=2-D array (concatenate along first dimension)
  To Workspace1 : ToWorkspace  VariableName=Days  SampleTime=1
      settings: Save2DSignal=2-D array (concatenate along first dimension)
  To Workspace2 : ToWorkspace  VariableName=Work_speed  SampleTime=1
      settings: Save2DSignal=2-D array (concatenate along first dimension)
  To Workspace3 : ToWorkspace  VariableName=OptSpring  SampleTime=-1
      settings: Decimation=10  Save2DSignal=2-D array (concatenate along first dimension)
  To Workspace4 : ToWorkspace  VariableName=OptFall  SampleTime=-1
      settings: Decimation=10  Save2DSignal=2-D array (concatenate along first dimension)
  "conv to ha (1000 m2 to 10000m2) " : Gain  Gain=0.1
  conv to ha (1000 m2 to 10000m2) 1 : Constant  Value=0.1
  "hours to days " : Gain  Gain=1/24
  hours to days 1 : Gain  Gain=1/24
  hours to days 2 : Gain  Gain=1/24
  Out2 : Outport  VectorParamsAs1DForOutWhenUnconnected=off
  Out3 : Outport  Port=2  VectorParamsAs1DForOutWhenUnconnected=off
  Out4 : Outport  Port=3  VectorParamsAs1DForOutWhenUnconnected=off
  Out5 : Outport  Port=4  VectorParamsAs1DForOutWhenUnconnected=off
  tag scope: FieldSize=global, HectEnt=global, WorkTemp=global, X=global
  wires:
  [Field_size_matrix] -> Chart/1(FieldSize)
  Chart/1(X) -> Memory/1
  [v] -> Constant values/2
  [EstBat] -> Constant values/1
  [field_eff] -> Constant values/3
  Constant values/1 -> "conv to ha (1000 m2 to 10000m2) "/1
  "conv to ha (1000 m2 to 10000m2) "/1 -> [HectEnt], HectaresPerEnt [ha/traktor]/1
  [H] -> Terminator/1
  Chart/2(GateControl) -> Out2/1
  Chart/3(N) -> Scope2/2, Memory1/1
  Chart/4(H_out) -> Out5/1
  Memory1/1 -> Out3/1
  [P_fieldwork] -> Constant values/5
  [W_fieldwork] -> Constant values/4
  Clock/1 -> Chart/2(T)
  [X_1] -> Chart/3(X_1)
  [X_2] -> Chart/4(X_2)
  [X_3] -> Chart/5(X_3)
  [N_max] -> Chart/6(N_max)
  N_block/1 -> Chart/7(N_Block)
  Chart/5(Size) -> [FieldSize], Scope2/3
  Chart/6(T_1) -> Add/1
  Chart/7(T_2) -> Add/2
  Chart/8(T_3) -> Add/3
  Add/1 -> Add1/2
  Clock1/1 -> Add1/1
  Add1/1 -> Divide/1
  Constant/1 -> Divide/2
  Divide/1 -> To Workspace1/1, Days required/1
  [X_val] -> Chart/8(X_val)
  Chart/9(Time) -> "hours to days "/1
  "hours to days "/1 -> To Workspace/1
  conv to ha (1000 m2 to 10000m2) 1/1 -> Constant values1/4
  [W_fieldwork] -> Constant values1/3
  [field_eff] -> Constant values1/2
  [v] -> Constant values1/1
  Constant values1/1 -> Chart/9(WorkSpeed), To Workspace2/1
  Chart/10(WorkOut) -> Integrator/1
  Integrator/1 -> Memory2/1, Scope/2  "WorkOut"
  Memory2/1 -> Chart/10(WorkIn)
  Chart/11(WorkTemp) -> [WorkTemp], Scope/3  "Ha worked per field"
  [X_val] -> Scope2/1
  [State] -> Scope2/5
  [WorkTemp] -> Scope2/4
  [FieldSize] -> Scope/1  "Field size"
  [Workability] -> Chart/11(Workability)
  Chart/12(TimeSpring) -> hours to days 1/1
  Chart/13(TimeFall) -> hours to days 2/1
  hours to days 1/1 -> Display/1, To Workspace3/1
  hours to days 2/1 -> Display1/1, To Workspace4/1
  Memory/1 -> [X], Out4/1

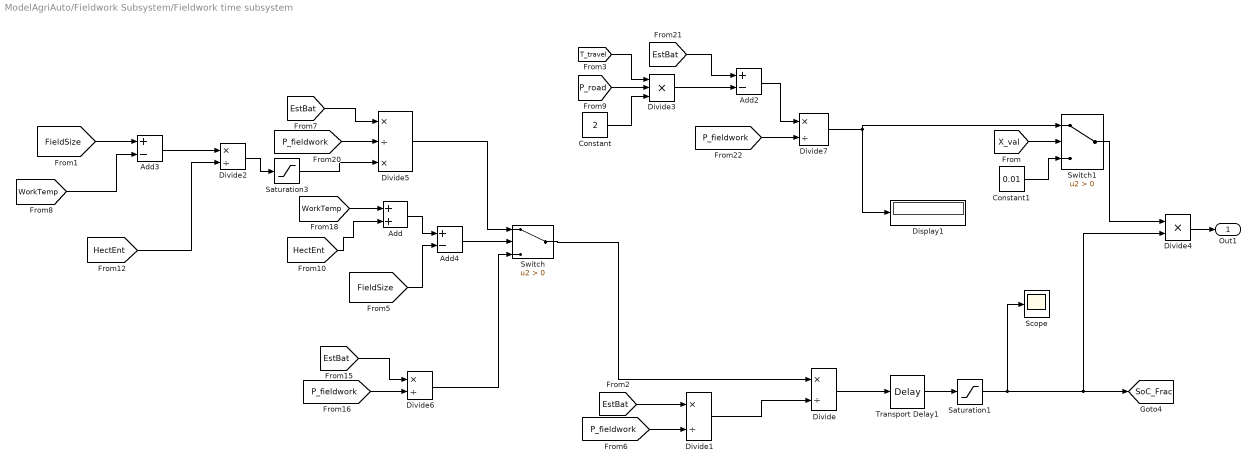
== system ModelAgriAuto/Fieldwork Subsystem/Fieldwork time subsystem  ==
  Add : Sum
  Add2 : Sum  Inputs=+-
  Add3 : Sum  Inputs=+-
  Add4 : Sum  Inputs=+-
  Constant : Constant  Value=2
  Constant1 : Constant  Value=0.01
  Display1 : Display
  Divide{,1..2,6..7} (5 alike) : Product  Inputs=*/
  Divide3 : Product  Inputs=***
  Divide4 : Product  Inputs=**
  Divide5 : Product  Inputs=*/*
  Saturation1 : Saturate  UpperLimit=1  LowerLimit=0.2
  Saturation3 : Saturate  UpperLimit=inf  LowerLimit=0
  Scope : Scope
  Switch : Switch  Criteria=u2 > Threshold  SaturateOnIntegerOverflow=off  InputSameDT=off
  Switch1 : Switch  Criteria=u2 > Threshold  SaturateOnIntegerOverflow=off  InputSameDT=off
  Transport Delay1 : TransportDelay  DelayTime=0.1  InitialOutput=0.1
  Out1 : Outport  VectorParamsAs1DForOutWhenUnconnected=off
  tag scope: SoC_Frac=global
  wires:
  [P_fieldwork] -> Divide6/2
  [FieldSize] -> Add4/2
  Add/1 -> Add4/1
  [WorkTemp] -> Add/1
  Add4/1 -> Switch/2
  [HectEnt] -> Add/2
  Divide6/1 -> Switch/3
  Switch/1 -> Divide/1
  [P_fieldwork] -> Divide1/2
  Divide1/1 -> Divide/2
  [EstBat] -> Divide1/1
  Transport Delay1/1 -> Saturation1/1
  Divide/1 -> Transport Delay1/1
  Saturation1/1 -> Scope/1, Divide4/2, [SoC_Frac]
  [FieldSize] -> Add3/1
  [WorkTemp] -> Add3/2
  Add3/1 -> Divide2/1
  Divide2/1 -> Saturation3/1
  Saturation3/1 -> Divide5/3
  [EstBat] -> Divide5/1
  [P_fieldwork] -> Divide5/2
  [EstBat] -> Divide6/1
  [P_fieldwork] -> Divide7/2
  Divide5/1 -> Switch/1
  Divide7/1 -> Display1/1, Switch1/1
  [HectEnt] -> Divide2/2
  [P_road] -> Divide3/2
  [T_travel] -> Divide3/1
  Constant/1 -> Divide3/3
  [X_val] -> Switch1/2
  Switch1/1 -> Divide4/1
  Constant1/1 -> Switch1/3
  Divide4/1 -> Out1/1
  Divide3/1 -> Add2/2
  [EstBat] -> Add2/1
  Add2/1 -> Divide7/1

== system ModelAgriAuto/Inputs & Data/Battery and driveline inputs ==
  note: Efficiency of the Driveline
  "\"Useful Battery Capacity\"" : Product  Inputs=5
  Battery capacity reduction : Subsystem
  Constant : Constant
  Constant1 : Constant  Value=Degradation
  Multiport Switch : MultiPortSwitch  Inputs=2  SaturateOnIntegerOverflow=off  InputSameDT=off
  To Workspace1 : ToWorkspace  VariableName=SOC  SampleTime=10
      settings: Decimation=10  Save2DSignal=2-D array (concatenate along first dimension)
  "Total Transmission Efficiency " : Constant  Value=0.85
  omegaRoadGear1 : Product  Inputs=**
  tag scope: Battery_size=global, EMeff=global, EstBat=global, P_Vehicle=global
  wires:
  [BATeff] -> "\"Useful Battery Capacity\""/4
  [EMeff] -> "\"Useful Battery Capacity\""/2
  "\"Useful Battery Capacity\""/1 -> [EstBat]
  [Battery] -> "\"Useful Battery Capacity\""/1, [Battery_size]
  [SOC] -> "\"Useful Battery Capacity\""/3
  [Power] -> [P_Vehicle]
  omegaRoadGear1/1 -> [EMeff]
  "Total Transmission Efficiency "/1 -> omegaRoadGear1/2
  [MotorEff] -> omegaRoadGear1/1
  Battery capacity reduction/1(Out1) -> Multiport Switch/3
  Constant/1 -> Multiport Switch/2
  Multiport Switch/1 -> To Workspace1/1, "\"Useful Battery Capacity\""/5
  Constant1/1 -> Multiport Switch/1

== system ModelAgriAuto/Inputs & Data/Charging inputs ==
  tag scope: P_charger=global, P_charger_swap=global
  wires:
  [Charger] -> [P_charger]
  [Charger] -> [P_charger_swap]

== system ModelAgriAuto/Inputs & Data/Field inputs ==
  Crop on field : Constant  Value="[1 4 2 2 3 1  4 1 3 4 2 3]"
  Distance field-farm [km] : Constant  Value=[DField DField DField DField DField DField DField DField DField DField DField DField]
  Distance field-farm [km]1 : Constant  Value=[1 1 2 2 3 3 4 4 5 5 6 6]
  Field efficiancy : Subsystem
  Field forces : Subsystem
  Field sizes [ha] : Constant  Value=[10 16 20 13 15 26 6 14 22 28 17 13]
  Fieldwork choice & data : Subsystem
  Sum of Elements : Sum  Inputs=+
  Switch : Switch  Criteria=u2 > Threshold  SaturateOnIntegerOverflow=off  InputSameDT=off
  Width : Width
  tag scope: Field_distance=global, Field_size_matrix=global, H=global, N_max=global, Rotation_choice=global
  wires:
  Field sizes [ha]/1 -> Width/1, Sum of Elements/1, [Field_size_matrix]
  Sum of Elements/1 -> [H]
  Crop on field/1 -> [Rotation_choice]
  Switch/1 -> [Field_distance]
  Distance field-farm [km]1/1 -> Switch/3
  Distance field-farm [km]/1 -> Switch/2, Switch/1
  Width/1 -> [N_max]

== system ModelAgriAuto/Inputs & Data/Fuel//mode selection  ==
  note: Battery/Tank efficiency
  note: State of charge - usable fraction of energy reservoir
  note: Charger efficiency, fraction
  note: Charger choice, list
  note: Motor efficiency, fraction
  note: 1=CC, 2=BES, 3=Diesel, 4=H2
  " " : Constant  Value=0.95
  BatteryEfficiency : Constant  Value=0.97
  BatteryEfficiency1 : Constant  Value=0.97
  BatteryEfficiency2 : Constant
  Charger eff 1 : Constant  Value=0.95
  Constant{,1,6..7,9..12} (8 alike) : Constant
  Constant2 : Constant  Value=2
  Constant3 : Constant  Value=0.95
  Constant4 : Constant  Value=0.95
  Constant5 : Constant  Value=0.3
  Constant8 : Constant  Value=0.6
  Multiport Switch{,1..4} (5 alike) : MultiPortSwitch  Inputs=4  SaturateOnIntegerOverflow=off  InputSameDT=off
  "Useable SoC " : Constant  Value=0.8
  Useable SoC 1 : Constant  Value=0.8
  tag scope: BATeff=global, ChargerChoice=global, Charger_eff=global, MotorEff=global, SOC=global
  wires:
  [Fuel] -> Multiport Switch/1
  [Fuel] -> Multiport Switch2/1
  [Fuel] -> Multiport Switch3/1
  Constant/1 -> Multiport Switch/2
  Constant1/1 -> Multiport Switch/4
  Constant2/1 -> Multiport Switch/3
  Multiport Switch/1 -> [ChargerChoice]
  Multiport Switch3/1 -> [MotorEff]
  Constant3/1 -> Multiport Switch3/2
  Constant4/1 -> Multiport Switch3/3
  Constant5/1 -> Multiport Switch3/4
  " "/1 -> Multiport Switch2/2
  Multiport Switch2/1 -> [Charger_eff]
  Charger eff 1/1 -> Multiport Switch2/3
  Constant6/1 -> Multiport Switch2/4
  Constant7/1 -> Multiport Switch/5
  Constant8/1 -> Multiport Switch3/5
  Constant9/1 -> Multiport Switch2/5
  [Fuel] -> Multiport Switch1/1
  "Useable SoC "/1 -> Multiport Switch1/2
  Useable SoC 1/1 -> Multiport Switch1/3
  Constant11/1 -> Multiport Switch1/5
  Constant10/1 -> Multiport Switch1/4
  Multiport Switch1/1 -> [SOC]
  [Fuel] -> Multiport Switch4/1
  Multiport Switch4/1 -> [BATeff]
  BatteryEfficiency/1 -> Multiport Switch4/2
  BatteryEfficiency1/1 -> Multiport Switch4/3
  Constant12/1 -> Multiport Switch4/4
  BatteryEfficiency2/1 -> Multiport Switch4/5
